simulink model "temp"  (R2024b)
settings: Solver=VariableStepAuto  StartTime=0.0  StopTime=10.0  RelTol=1e-3
libraries: simulink x1
settings Model: Creator=Arhaan  LastModifiedBy=Arhaan

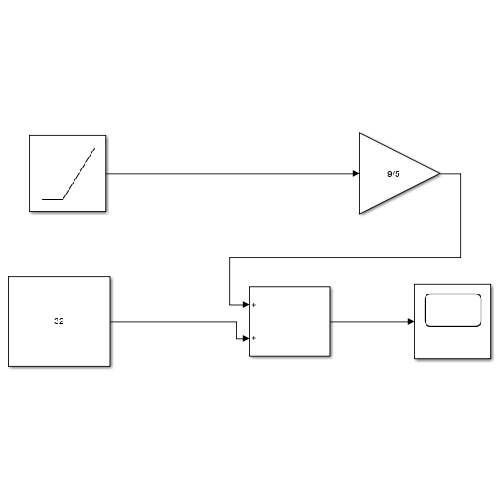
[thumbnail: Simulink's stored preview of the top-level diagram]
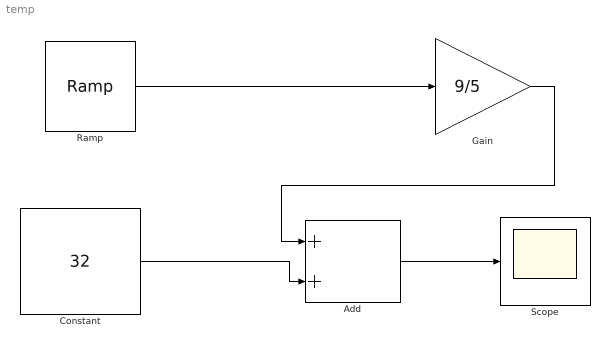
== system temp ==
  Add : Sum
  Constant : Constant  Value=32
  Gain : Gain  Gain=9/5
  Ramp : simulink/Sources/Ramp  slope=1  start=0  InitialOutput=0
  Scope : Scope
  wires:
  Ramp/1 -> Gain/1
  Gain/1 -> Add/1
  Constant/1 -> Add/2
  Add/1 -> Scope/1
